simulink model "cordic_cosim"  (Simulink 6.4)
settings: Solver=FixedStepDiscrete  SolverMode=SingleTasking  StartTime=0.0  StopTime=12e-2  RelTol=1e-3
libraries: modelsimlib x1, simulink x1
settings Model: LastModifiedBy=Administrador

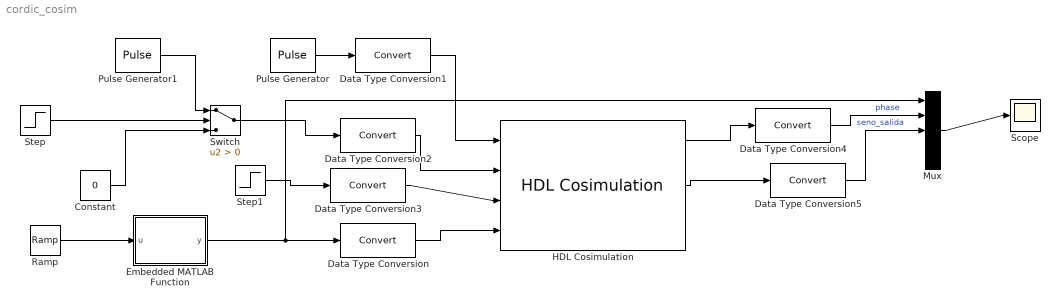
== system cordic_cosim ==
  Constant : Constant  Value=0  OutDataType=sfix(16)  ConRadixGroup=Use specified scaling  OutScaling=2^0  SampleTime=-1  FramePeriod=inf
  Data Type Conversion : DataTypeConversion  OutDataTypeMode=Specify via dialog  OutScaling=2^(-10)  RndMeth=Nearest  SampleTime=1e-5  SaturateOnIntegerOverflow=on
  Data Type Conversion1 : DataTypeConversion  OutDataTypeMode=boolean
  Data Type Conversion2 : DataTypeConversion  OutDataTypeMode=boolean
  Data Type Conversion3 : DataTypeConversion  OutDataTypeMode=boolean
  Data Type Conversion4 : DataTypeConversion
  Data Type Conversion5 : DataTypeConversion
  Embedded MATLAB Function : Stateflow chart
  HDL Cosimulation : modelsimlib/HDL Cosimulation  DialogController=modelsimddg.CoSim  DialogControllerArgs=DataTag0  PortPaths=/cordic/clk;/cordic/run;/cordic/rst;/cordic/angle;/cordic/sin;/cordic/cos;/cordic/done  PortModes=[1 1 1 1 2 2 2 ]  PortTimes=[1,1,1,1,1e-5,1e-5,1e-5]  PortSigns=[-1 -1 -1 -1 1 1 -1 ]  PortFracLengths=[0,0,0,0,10,10,10]  CommLocal=on  CommSharedMemory=off  CommPortNumber=4449  CommShowInfo=on  ClockModes=[]  ClockTimes=[]  TclPreSimCommand="echo \"Running Simulink Cosimulation block.\""  TclPostSimCommand="echo \"done\""  TimingMode=s  TimingScaleFactor=1  idxCellArray={'UNUSED_VAR'}
  Mux : Mux  Inputs=5
  Pulse Generator : DiscretePulseGenerator  PulseType=Time based  Period=1/(1e6)  PulseWidth=50
  Pulse Generator1 : DiscretePulseGenerator  PulseType=Time based  Period=0.1e-3  PulseWidth=2
  Ramp : simulink/Sources/Ramp  SystemSampleTime=-1  slope=2*pi*50  start=0  X0=0
  Scope : Scope
      settings: YMin=-3.25  YMax=2.25  MaxDataPoints=500000
  Step : Step  Time=4*(1/1e6)
  Step1 : Step  Time=6*(1/1e6)  Before=1  After=0
  Switch : Switch  Criteria=u2 > Threshold  RndMeth=Nearest  ZeroCross=off  SampleTime=1e-7
  wires:
  Data Type Conversion/1 -> HDL Cosimulation/4
  Embedded MATLAB Function/1(y) -> Data Type Conversion/1, Mux/1
  Pulse Generator/1 -> Data Type Conversion1/1
  Data Type Conversion1/1 -> HDL Cosimulation/1
  Switch/1 -> Data Type Conversion2/1
  Data Type Conversion2/1 -> HDL Cosimulation/2
  Step1/1 -> Data Type Conversion3/1
  Data Type Conversion3/1 -> HDL Cosimulation/3
  Constant/1 -> Switch/3
  Step/1 -> Switch/2
  Pulse Generator1/1 -> Switch/1
  Mux/1 -> Scope/1
  HDL Cosimulation/1 -> Data Type Conversion4/1
  Data Type Conversion4/1 -> Mux/2  "phase"
  HDL Cosimulation/2 -> Data Type Conversion5/1
  Data Type Conversion5/1 -> Mux/3  "seno_salida"
  Ramp/1 -> Embedded MATLAB Function/1(u)

== matlab function Embedded MATLAB Function ==
  data: u input inherited; y output inherited
function y = fcn(u)
% This block supports an embeddable subset of the MATLAB language.
% See the help menu for details. 

y = mod(u,2*pi) - pi;
